simulink model "CruiseControl_DivByZero"  (R2021a)
settings: Solver=FixedStepDiscrete  StartTime=0.0  StopTime=16  FixedStep=0.1  RelTol=1e-3  EnableMultiTasking=on
PreLoadFcn:
  | CruiseControl_DivByZero_dd;
values from neighbouring files (symbols this model uses):
  holdrate = mpt.Parameter    [CruiseControl_DivByZero_dd.m]    (also in CruiseControl_dd.sldd = 5.0
                
                    
                  )
  incdec = mpt.Parameter    [CruiseControl_DivByZero_dd.m]    (also in CruiseControl_dd.sldd = 1.0
                
                    
                  )
  maxtspeed = mpt.Parameter    [CruiseControl_DivByZero_dd.m]    (also in CruiseControl_dd.sldd = 90.0
                
                    
                 )
  mintspeed = mpt.Parameter    [CruiseControl_DivByZero_dd.m]    (also in CruiseControl_dd.sldd = 20.0
                
                    
                 )
settings Model: Creator=The MathWorks Inc.  LastModifiedBy=patcanny
settings SolverCC: AlgebraicLoopSolver=TrustRegion
settings DataIOCC: LimitDataPoints=on  SaveFormat=Array  SaveOutput=off  SaveTime=off  ReturnWorkspaceOutputs=off
settings OptimizationCC: DefaultParameterBehavior=Inlined  InlineInvariantSignals=on  ExpressionDepthLimit=2147483647  InitFltsAndDblsToZero=on  LifeSpan=inf  EfficientTunableParamExpr=on
settings DebuggingCC: SaveWithParameterizedLinksMsg=none  SolverPrmCheckMsg=warning  StateNameClashWarn=warning  StrictBusMsg=ErrorOnBusTreatedAsVector  SFUnexpectedBacktrackingDiag=warning  SFNoUnconditionalDefaultTransitionDiag=warning  SFExecutionAtInitializationDiag=none  SFMachineParentedDataDiag=warning  ArithmeticOperatorsInVariantConditions=warning
settings HardwareCC: ProdBitPerPointer=32  ProdBitPerSizeT=32  ProdBitPerPtrDiffT=32  ProdLargestAtomicFloat=None  ProdIntDivRoundTo=Undefined  ProdEndianess=Unspecified  ProdWordSize=32  ProdHWDeviceType=32-bit Generic
settings ModelReferenceCC: ModelReferenceNumInstancesAllowed=Single  PropagateSignalLabelsOutOfModel=off
settings SFSimCC: SimUseLocalCustomCode=off  SimParseCustomCode=off  MATLABDynamicMemAlloc=off  CustomCodeUndefinedFunction=UseInterfaceOnly
settings RTWCC: SystemTargetFile=ert.tlc  GenCodeOnly=on  TemplateMakefile=ert_default_tmf  GenerateReport=on  RTWUseLocalCustomCode=off  IncludeHyperlinkInReport=on  LaunchReport=on  PortableWordSizes=on  GenerateTraceInfo=on  GenerateTraceReport=on  GenerateTraceReportSl=on  GenerateTraceReportSf=on  GenerateTraceReportEml=on
settings CodeAppCC: IgnoreCustomStorageClasses=off  StateflowObjectComments=on
settings ERTTargetCC: MultiwordLength=2048  GenerateSampleERTMain=on  InlinedParameterPlacement=NonHierarchical  ERTCustomFileTemplate=example_file_process.tlc  ConvertIfToSwitch=off  SuppressUnreachableDefaultCases=off
settings ConfigComp: CovEnable=on  CovScope=ReferencedModels  RecordCoverage=on  CovMetricSettings=dcme  CovExternalEMLEnable=off  CovSFcnEnable=off  DVMode=DesignErrorDetection  DVMaxProcessTime=3000  DVAutomaticStubbing=off  DVMakeOutputFilesUnique=off  DVParameters=on  DVParametersUseConfig=on  DVModelCoverageObjectives=MCDC  DVMaxTestCaseSteps=500  DVTestSuiteOptimization=CombinedObjectives  DVAssertions=EnableAll  DVProofAssumptions=EnableAll  DVIgnoreCovSatisfied=on  DVCoverageDataFile=CruiseControlCovManual.cvt  DVDetectActiveLogic=on  DVDetectIntegerOverflow=off  DVMaxViolationSteps=50  DVReportIncludeGraphics=on

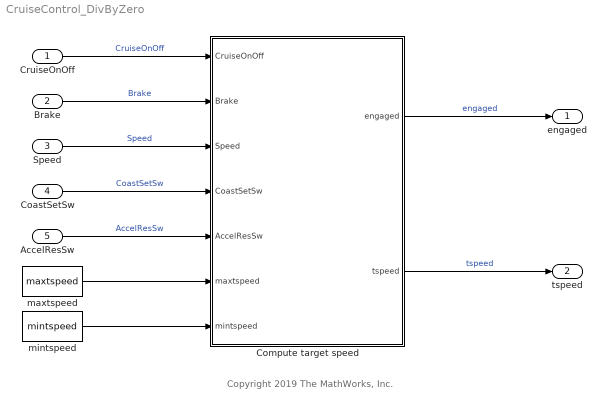
== system CruiseControl_DivByZero ==
  note: Copyright 2019 The MathWorks, Inc.
  CruiseOnOff : Inport  PortDimensions=1
  Brake : Inport  Port=2  PortDimensions=1
  Speed : Inport  Port=3  PortDimensions=1
  CoastSetSw : Inport  Port=4  PortDimensions=1
  AccelResSw : Inport  Port=5  PortDimensions=1
  Compute target speed : Stateflow chart  TreatAsAtomicUnit=on
  maxtspeed : Constant  Value=maxtspeed  SampleTime=-1
  mintspeed : Constant  Value=mintspeed  SampleTime=-1
  engaged : Outport  VectorParamsAs1DForOutWhenUnconnected=off
  tspeed : Outport  Port=2  VectorParamsAs1DForOutWhenUnconnected=off
  wires:
  Compute target speed/2(tspeed) -> tspeed/1  "tspeed"
  Compute target speed/1(engaged) -> engaged/1  "engaged"
  AccelResSw/1 -> Compute target speed/5(AccelResSw)  "AccelResSw"
  CruiseOnOff/1 -> Compute target speed/1(CruiseOnOff)  "CruiseOnOff"
  Brake/1 -> Compute target speed/2(Brake)  "Brake"
  CoastSetSw/1 -> Compute target speed/4(CoastSetSw)  "CoastSetSw"
  Speed/1 -> Compute target speed/3(Speed)  "Speed"
  maxtspeed/1 -> Compute target speed/6(maxtspeed)
  mintspeed/1 -> Compute target speed/7(mintspeed)

== stateflow chart CruiseControl_DivByZero/Compute target speed ==
  state OFF
    en:
    engaged = false;
    tspeed = 0;
  state CRUISE
    state ON
      en: engaged = true;
      state Accel
        entry: tspeed = tspeed + incdec;
      state Steady
      state Coast
        entry: tspeed = tspeed - incdec;
      (junction 60) -> Accel
      (junction 57) -> (junction 60) : [after(incdec*10/holdrate,tick)]
      Accel -> (junction 57) [order 2]
      Steady -> Accel [order 1] : [hasChangedTo(AccelResSw,true) ...
          | && tspeed < maxtspeed]
      Accel -> Steady [order 1] : [!AccelResSw || ...
          | tspeed > maxtspeed]
      Steady -> (junction 75) [order 3] : [hasChangedTo(CoastSetSw,true)]
      (default) -> (junction 75)
      (junction 75) -> (junction 77) : {tspeed = Speed;}
      (junction 77) -> Steady
      Steady -> Coast [order 2] : [hasChangedTo(CoastSetSw,true) ...
          | && tspeed > mintspeed]
      Coast -> Steady [order 1] : [!CoastSetSw || ...
          | tspeed < mintspeed]
      (junction 72) -> Coast
      (junction 71) -> (junction 72) : [after(incdec*10/holdrate,tick)]
      Coast -> (junction 71) [order 2]
    state STANDBY
      en:
      engaged=false;
    (default) -> STANDBY
    ON -> STANDBY : [Brake||Speed> maxtspeed||Speed<mintspeed]
    STANDBY -> (junction 103) : [~Brake && ...
        | Speed<=maxtspeed && ...
        | Speed>=mintspeed]
    (junction 103) -> Steady [order 1] : [hasChangedTo(AccelResSw,true)...
        | &&tspeed!=0]
    (junction 103) -> (junction 106) [order 2]
    (junction 106) -> ON : [hasChangedTo(CoastSetSw,true)]
  (default) -> OFF
  OFF -> CRUISE : [CruiseOnOff]
  CRUISE -> OFF : [~CruiseOnOff]
  data: engaged output boolean; CruiseOnOff input; Brake input; Speed input; CoastSetSw input; AccelResSw input; tspeed output single; incdec parameter; holdrate parameter; maxtspeed input; mintspeed input
  events: CruiseDiseng local FUNCTION_CALL_EVENT; CruiseEng local FUNCTION_CALL_EVENT
